simulink model "lqr_ydx01"  (R2022b)
settings: Solver=VariableStepAuto  StartTime=0.0  StopTime=70  RelTol=1e-3
values from neighbouring files (symbols this model uses):
  cx = 0:0.1:120    [lqrydx_ref_01.m]
  cy = dy1/2.*(1+tanh(z1))-dy2/2.*(1+tanh(z2))    [lqrydx_ref_01.m]
  r_k = abs(dd_y) ./ (1+d_y.^2).^(3/2)    [lqrydx_ref_01.m]
  r_yaw = atan2(dif_yyyy , dif_xxxx)    [lqrydx_ref_01.m]
libraries: Solver_SF x2, simulink x2
settings Model: Creator=wenju  LastModifiedBy=admin
settings ModelReferenceCC: EnableRefExpFcnMdlSchedulingChecks=on

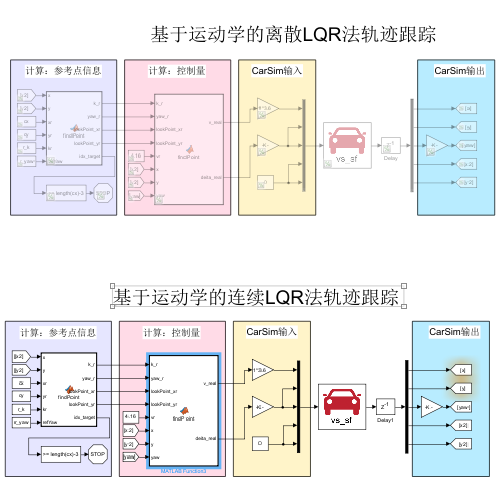
[thumbnail: Simulink's stored preview of the top-level diagram]
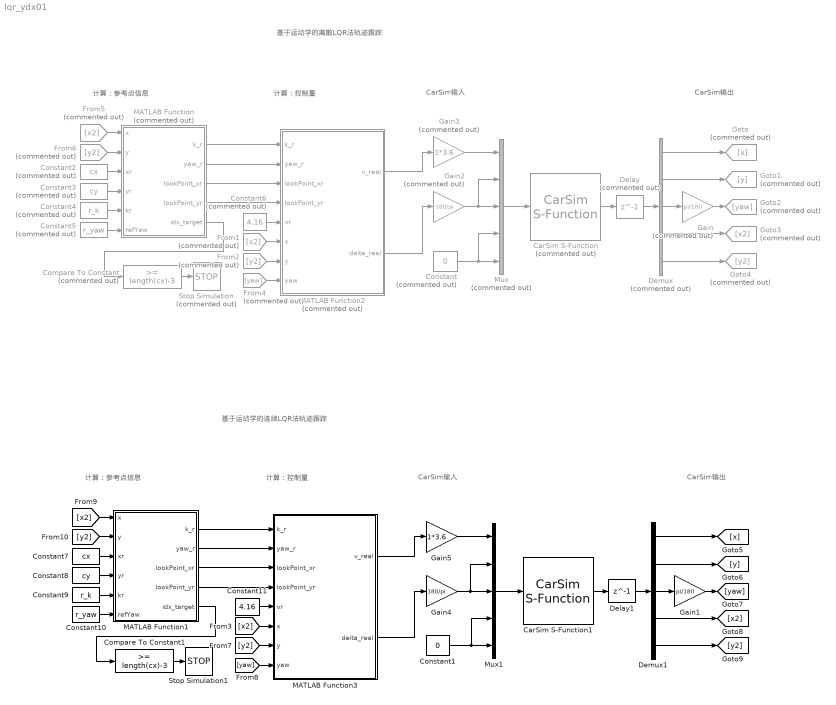
== system lqr_ydx01 ==
  note: CarSim输出
  note: 基于运动学的离散LQR法轨迹跟踪
  note: CarSim输入
  note: 计算：参考点信息
  note: 计算：控制量
  note: CarSim输出
  note: 计算：参考点信息
  note: CarSim输入
  note: 计算：控制量
  note: 基于运动学的连续LQR法轨迹跟踪
  CarSim S-Function : Solver_SF/CarSim S-Function  Priority=1  Commented=on  SIMFILE=simfile.sim  Run_RTs=off  vs_state_ind=Run  StopMode_ind=Vehicle Model
  CarSim S-Function1 : Solver_SF/CarSim S-Function  Priority=1  SIMFILE=simfile.sim  Run_RTs=off  vs_state_ind=Run  StopMode_ind=Vehicle Model
  Compare To Constant : simulink/Logic and Bit Operations/Compare To Constant  Commented=on  relop=>=  const=length(cx)-3  OutDataTypeStr=boolean
  Compare To Constant1 : simulink/Logic and Bit Operations/Compare To Constant  relop=>=  const=length(cx)-3  OutDataTypeStr=boolean
  Constant : Constant  Commented=on  Value=0
  Constant1 : Constant  Value=0
  Constant10 : Constant  Value=r_yaw
  Constant11 : Constant  Value=4.16
  Constant2 : Constant  Commented=on  Value=cx
  Constant3 : Constant  Commented=on  Value=cy
  Constant4 : Constant  Commented=on  Value=r_k
  Constant5 : Constant  Commented=on  Value=r_yaw
  Constant6 : Constant  Commented=on  Value=4.16
  Constant7 : Constant  Value=cx
  Constant8 : Constant  Value=cy
  Constant9 : Constant  Value=r_k
  Delay : Delay  Commented=on  DelayLength=1  InitialCondition=0  UseCircularBuffer=on
  Delay1 : Delay  DelayLength=1  InitialCondition=0  UseCircularBuffer=on
  Demux : Demux  Commented=on  Outputs=5
  Demux1 : Demux  Outputs=5
  From1 : From  Commented=on  GotoTag=x2
  From2 : From  Commented=on  GotoTag=y2
  From4 : From  Commented=on  GotoTag=yaw
  From5 : From  Commented=on  GotoTag=x2
  From6 : From  Commented=on  GotoTag=y2
  Gain : Gain  Commented=on  Gain=pi/180
  Gain1 : Gain  Gain=pi/180
  Gain2 : Gain  Commented=on  Gain=180/pi
  Gain3 : Gain  Commented=on  Gain=1*3.6
  Gain4 : Gain  Gain=180/pi
  Gain5 : Gain  Gain=1*3.6
  Goto : Goto  Commented=on  GotoTag=x
  Goto1 : Goto  Commented=on  GotoTag=y
  Goto2 : Goto  Commented=on  GotoTag=yaw
  Goto3 : Goto  Commented=on  GotoTag=x2
  Goto4 : Goto  Commented=on  GotoTag=y2
  MATLAB Function : MATLAB Function  Commented=on  TreatAsAtomicUnit=on
  MATLAB Function1 : MATLAB Function  TreatAsAtomicUnit=on
  MATLAB Function2 : MATLAB Function  Commented=on  TreatAsAtomicUnit=on
  MATLAB Function3 : MATLAB Function  TreatAsAtomicUnit=on
  Mux : Mux  Commented=on  Inputs=5
  Mux1 : Mux  Inputs=5
  Stop Simulation : Stop  Commented=on
  Stop Simulation1 : Stop
  wires:
  Mux/1 -> CarSim S-Function/1
  CarSim S-Function/1 -> Delay/1
  Delay/1 -> Demux/1
  Demux/1 -> Goto/1
  Demux/2 -> Goto1/1
  Demux/3 -> Gain/1
  Gain/1 -> Goto2/1
  Constant/1 -> Mux/4, Mux/5
  Gain2/1 -> Mux/2, Mux/3
  Gain3/1 -> Mux/1
  Constant2/1 -> MATLAB Function/3(xr)
  Constant3/1 -> MATLAB Function/4(yr)
  Constant4/1 -> MATLAB Function/5(kr)
  Constant5/1 -> MATLAB Function/6(refYaw)
  From4/1 -> MATLAB Function2/8(yaw)
  MATLAB Function/1(k_r) -> MATLAB Function2/1(k_r)
  MATLAB Function/2(yaw_r) -> MATLAB Function2/2(yaw_r)
  MATLAB Function/3(lookPoint_xr) -> MATLAB Function2/3(lookPoint_xr)
  MATLAB Function/4(lookPoint_yr) -> MATLAB Function2/4(lookPoint_yr)
  Constant6/1 -> MATLAB Function2/5(vr)
  MATLAB Function2/2(deita_real) -> Gain2/1
  MATLAB Function2/1(v_real) -> Gain3/1
  Compare To Constant/1 -> Stop Simulation/1
  MATLAB Function/5(idx_target) -> Compare To Constant/1
  Demux/4 -> Goto3/1
  Demux/5 -> Goto4/1
  From5/1 -> MATLAB Function/1(x)
  From6/1 -> MATLAB Function/2(y)
  From1/1 -> MATLAB Function2/6(x)
  From2/1 -> MATLAB Function2/7(y)
  Gain4/1 -> Mux1/2, Mux1/3
  MATLAB Function3/2(deita_real) -> Gain4/1
  Demux1/2 -> [y]
  MATLAB Function1/1(k_r) -> MATLAB Function3/1(k_r)
  Constant10/1 -> MATLAB Function1/6(refYaw)
  Constant1/1 -> Mux1/4, Mux1/5
  [y2] -> MATLAB Function3/7(y)
  CarSim S-Function1/1 -> Delay1/1
  [x2] -> MATLAB Function3/6(x)
  Compare To Constant1/1 -> Stop Simulation1/1
  [x2] -> MATLAB Function1/1(x)
  Constant11/1 -> MATLAB Function3/5(vr)
  Demux1/1 -> [x]
  Demux1/5 -> [y2]
  MATLAB Function1/5(idx_target) -> Compare To Constant1/1
  Constant7/1 -> MATLAB Function1/3(xr)
  Gain5/1 -> Mux1/1
  Constant8/1 -> MATLAB Function1/4(yr)
  Demux1/3 -> Gain1/1
  Demux1/4 -> [x2]
  Mux1/1 -> CarSim S-Function1/1
  MATLAB Function1/4(lookPoint_yr) -> MATLAB Function3/4(lookPoint_yr)
  [yaw] -> MATLAB Function3/8(yaw)
  MATLAB Function1/3(lookPoint_xr) -> MATLAB Function3/3(lookPoint_xr)
  Gain1/1 -> [yaw]
  Constant9/1 -> MATLAB Function1/5(kr)
  Delay1/1 -> Demux1/1
  MATLAB Function3/1(v_real) -> Gain5/1
  MATLAB Function1/2(yaw_r) -> MATLAB Function3/2(yaw_r)
  [y2] -> MATLAB Function1/2(y)

== matlab function lqr_ydx01/MATLAB Function1 ==
  data: k_r output; x input; yaw_r output; y input; xr input; yr input; kr input; refYaw input; lookPoint_xr output; lookPoint_yr output; idx_target output
% 首先在参考轨迹上搜索离当前车辆位置最近的点索引号，由索引号取出对应的参考量
function [k_r,yaw_r,lookPoint_xr, lookPoint_yr,idx_target] = findPoint(x,y, xr,yr,kr,refYaw)

% 找到距离当前位置最近的一个参考轨迹点的序号
n=length(xr);
d_min=(x-xr(1))^2+(y-yr(1))^2;
min=0;
for i = 1:n
    d = (x-xr(i))^2+(y-yr(i))^2; 
    if d<d_min
        d_min=d;
        min=i;
    end
end

% matlab 数组索引号从1开始，这里仿真matlab报错
if min<=1   
   min=1;
end

%由匹配点序号给出匹配点相关信息
idx_target = min;
lookPoint_xr = xr(idx_target);   %参考的x
lookPoint_yr = yr(idx_target);   %参考的y
k_r=kr(idx_target);              %参考的曲率，参考的前轮转角有参考曲率算出
yaw_r=refYaw(idx_target);        %参考的横摆角

end

== matlab function lqr_ydx01/MATLAB Function ==
  data: k_r output; x input; yaw_r output; y input; xr input; yr input; kr input; refYaw input; lookPoint_xr output; lookPoint_yr output; idx_target output
% 首先在参考轨迹上搜索离当前车辆位置最近的点索引号，由索引号取出对应的参考量
function [k_r,yaw_r,lookPoint_xr, lookPoint_yr,idx_target] = findPoint(x,y, xr,yr,kr,refYaw)

% 找到距离当前位置最近的一个参考轨迹点的序号
n=length(xr);
d_min=(x-xr(1))^2+(y-yr(1))^2;
min=0;
for i = 1:n
    d = (x-xr(i))^2+(y-yr(i))^2; 
    if d<d_min
        d_min=d;
        min=i;
    end
end

% matlab 数组索引号从1开始，这里仿真matlab报错
if min<=1   
   min=1;
end

%由匹配点序号给出匹配点相关信息
idx_target = min;
lookPoint_xr = xr(idx_target);   %参考的x
lookPoint_yr = yr(idx_target);   %参考的y
k_r=kr(idx_target);              %参考的曲率，参考的前轮转角有参考曲率算出
yaw_r=refYaw(idx_target);        %参考的横摆角

end

== matlab function lqr_ydx01/MATLAB Function2 ==
  data: k_r input; yaw_r input; lookPoint_xr input; lookPoint_yr input; vr input; x input; v_real output; y input; yaw input; deita_real output
% 首先在参考轨迹上搜索离当前车辆位置最近的点
function [v_real,deita_real] = findPoint(k_r,yaw_r,lookPoint_xr, lookPoint_yr,vr,x,y,yaw)

L=2.6;                           %车长
r_Delta = atan(L*k_r);           %参考的前轮转角，有固定公式

x_error  = x - lookPoint_xr;     %x方向误差
y_error = y - lookPoint_yr;      %y方向误差
yaw_error =  yaw - yaw_r;        %横摆角误差
e_X=[x_error;y_error;yaw_error]; %状态方程中的状态，即 x误差,y误差,横摆角误差

%% 离散状态空间方程：Xk+1=AXk+Buk 对应的矩阵
dt=0.05;                         %仿真步长
A = [1,  0,  -vr*dt*sin(yaw_r);
     0,  1,  vr * dt * cos(yaw_r);
     0,  0,  1];
B = [dt * cos(yaw_r),    0;
     dt * sin(yaw_r),    0;
     dt * tan(yaw_r)/L,  vr*dt/(L * cos(r_Delta)^2)];
%% 目标函数对应的Q,R矩阵设置
Q=[200,  0,  0;                  %权重矩阵Q
     0,  200,  0;
     0,  0,  80];

R=[7,  0;                        %权重矩阵R
     0,  20];

%% 求解P矩阵，稳住，按给定步骤求解即可
% 终止条件定义
iter_max = 500;                  %最大迭代次数
epsilon = 0.01;                  %允许误差

P_old = Q;
for i = 1:iter_max
    P_new = A' * P_old * A - (A' * P_old * B)/(R + B' * P_old * B) *( B' * P_old * A) +Q;
    if abs(P_new - P_old) <= epsilon
        break
    else
        P_old = P_new; 
    end
end

P = P_new;                       %最终P矩阵
%% 求得P矩阵后，根据公式，得到状态反馈增益K,并得到控制律
K = (B' * P * B + R) \ (B' * P * A);  
u = -K * e_X;                    %控制率，u=-kx，2行1列
%% 最终转换
v_delta = u(1);      
Delta_delta = u(2);

v_real=vr+v_delta;                  %最终控制量速度：V
deita_real=r_Delta+Delta_delta;     %最终控制量前轮转角：deita
end

== matlab function lqr_ydx01/MATLAB Function3 ==
  data: k_r input; yaw_r input; lookPoint_xr input; lookPoint_yr input; vr input; x input; v_real output; y input; yaw input; deita_real output
function [v_real,deita_real] = findPoint(k_r,yaw_r,lookPoint_xr, lookPoint_yr,vr,x,y,yaw)

L=2.6;                              %车长
r_Delta = atan(L*k_r);              %参考的前轮转角

x_error  = x - lookPoint_xr;        %x方向误差
y_error = y - lookPoint_yr;         %y方向误差
yaw_error =  yaw - yaw_r;           %横摆角误差
e_X=[x_error;y_error;yaw_error];    %状态方程中的状态

% X=AX+Bu 由状态方程系数矩阵
A = [0,  0,  -vr*sin(yaw_r);
     0,  0,  vr* cos(yaw_r);
     0,  0,  0];
B = [ cos(yaw_r),    0;
      sin(yaw_r),    0;
     tan(yaw_r)/L,  vr/(L * cos(r_Delta)^2)];

Q=[200,  0,  0;                     %权重矩阵Q
     0,  200,  0;
     0,  0,  80];
R=[7,  0;                           %权重矩阵R
     0,  20];

coder.extrinsic('lqr');             %此代码使在MATLAB function模块中可以使用求解工具lqr()
K=[ 0,    0,   0;
    0,    0,   0];
K = lqr(A,B,Q,R);                   %使用MATLAB工具求K

u = -K * e_X;                       %由反馈K得出最终控制量：u=-Kx

%控制律最终转换
v_delta = u(1);      
Delta_delta = u(2);
v_real=vr+v_delta;                  %最终控制量速度：V
deita_real=r_Delta+Delta_delta;     %最终控制量前轮转角：deita
end
